simulink model "Binary_Phase_Shift_Keying"  (R2023b)
settings: Solver=VariableStepAuto  StartTime=0.0  StopTime=10.0  RelTol=1e-3
libraries: commrandsrc3 x1
settings Model: Creator=online  LastModifiedBy=online

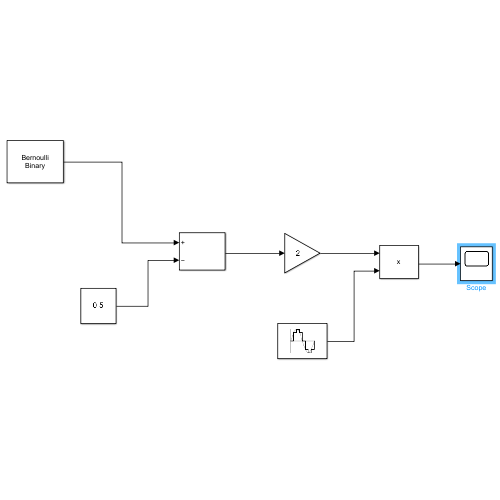
[thumbnail: Simulink's stored preview of the top-level diagram]
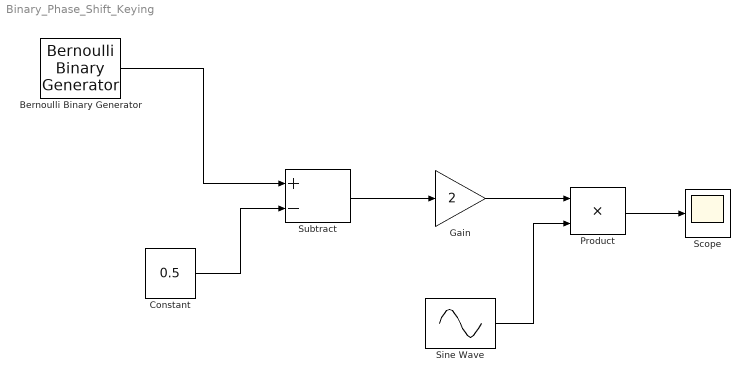
== system Binary_Phase_Shift_Keying ==
  Bernoulli Binary Generator : commrandsrc3/Bernoulli Binary Generator  ProbabilityOfZero=0.5  SeedSource=Auto  Seed=0  SampleTime=1  SamplesPerFrame=1  OutputDataType=double  SimulateUsing=Interpreted execution
  Constant : Constant  Value=0.5
  Gain : Gain  Gain=2
  Product : Product
  Scope : Scope
  Sine Wave : Sin  Frequency=4*pi  SampleTime=1/3200*pi
  Subtract : Sum  Inputs=+-
  wires:
  Bernoulli Binary Generator/1 -> Subtract/1
  Constant/1 -> Subtract/2
  Subtract/1 -> Gain/1
  Sine Wave/1 -> Product/2
  Gain/1 -> Product/1
  Product/1 -> Scope/1
